simulink model "Frequncy_measurement"  (Simulink 10.1)
settings: Solver=ode45  StartTime=0.0  StopTime=10  RelTol=1e-3  EnableMultiTasking=on
settings Model: Creator=Jayraj  LastModifiedBy=sebastian
settings DataIOCC: LimitDataPoints=on
settings DebuggingCC: UnderspecifiedInitializationDetection=Simplified  MergeDetectMultiDrivingBlocksExec=error
settings GRTTargetCC: CombineOutputUpdateFcns=on  GRTInterface=off

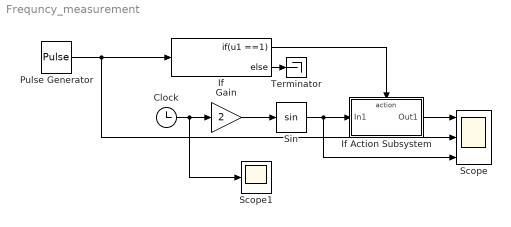
== system Frequncy_measurement ==
  Clock : Clock
  Gain : Gain  Gain=2
  If : If  IfExpression=u1 ==1
  If Action Subsystem : Subsystem  TreatAsAtomicUnit=on
  Pulse Generator : DiscretePulseGenerator  PulseType=Time based  PulseWidth=5
  Scope : Scope  NumInputPorts=3
  Scope1 : Scope
  Sin : Trigonometry
  Terminator : Terminator
  wires:
  Pulse Generator/1 -> Scope/2, If/1
  If/2 -> Terminator/1
  Clock/1 -> Scope1/1, Gain/1
  If/1 -> If Action Subsystem/Action
  If Action Subsystem/1(Out1) -> Scope/1
  Gain/1 -> Sin/1
  Sin/1 -> Scope/3, If Action Subsystem/1(In1)

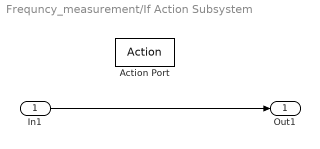
== system Frequncy_measurement/If Action Subsystem ==
  In1 : Inport
  Action Port : ActionPort  ActionPortLabel=if(u1 ==1)
  Out1 : Outport
  wires:
  In1/1 -> Out1/1
